simulink model "Shamit_jitesh"  (R2018a)
settings: Solver=VariableStepAuto  StartTime=0.0  StopTime=10.0  RelTol=1e-3
settings Model: Creator=shami  LastModifiedBy=shami

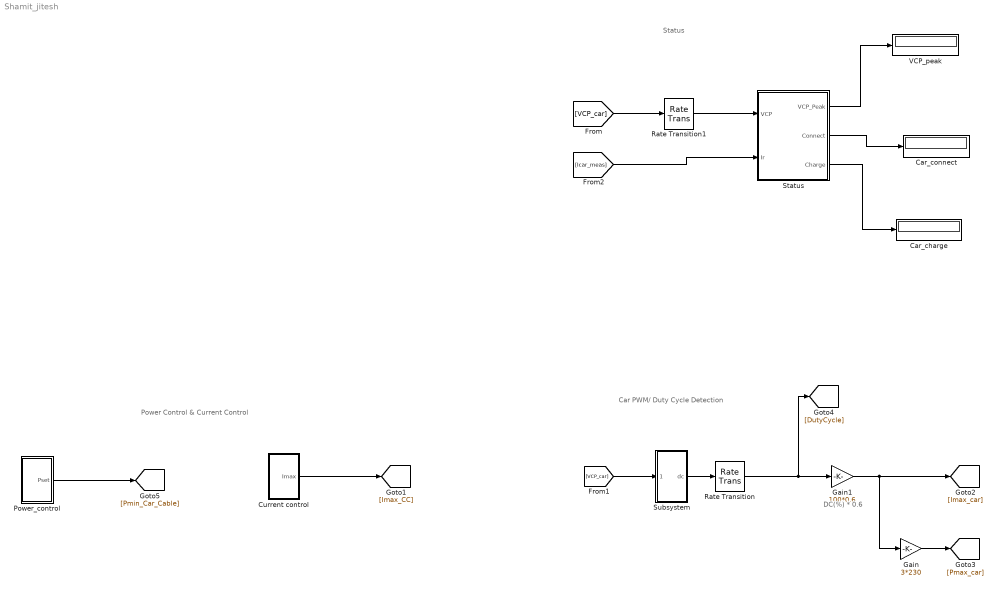
== system Shamit_jitesh ==
  note: Status
  note: Power Control & Current Control
  note: DC(%) * 0.6
  note: Car PWM/ Duty Cycle Detection
  Car_charge : Display
  Car_connect : Display
  Current control : Subsystem
  Gain : Gain  Gain=3*230
  Gain1 : Gain  Gain=100*0.6
  Power_control : Subsystem
  Rate Transition : RateTransition
  Rate Transition1 : RateTransition
  Status : Subsystem
  Subsystem : Subsystem
  VCP_peak : Display
  wires:
  Gain/1 -> [Pmax_car]
  Gain1/1 -> [Imax_car], Gain/1
  [VCP_car] -> Subsystem/1(pwm)
  Subsystem/1(dc) -> Rate Transition/1
  Rate Transition/1 -> [DutyCycle], Gain1/1
  Current control/1(Imax) -> [Imax_CC]
  Power_control/1(Pset) -> [Pmin_Car_Cable]
  [VCP_car] -> Rate Transition1/1
  Status/3("Charge ") -> Car_charge/1
  Status/1(VCP_Peak) -> VCP_peak/1
  [Icar_meas] -> Status/2(Ir)
  Status/2("Connect ") -> Car_connect/1
  Rate Transition1/1 -> Status/1(VCP)

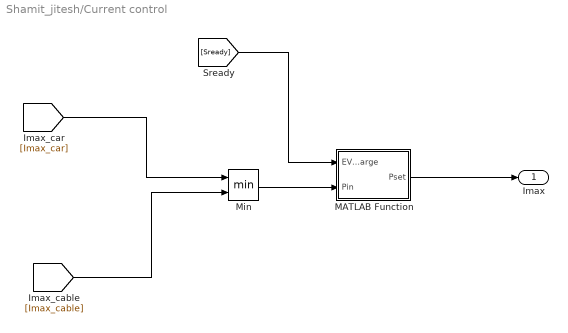
== system Shamit_jitesh/Current control ==
  MATLAB Function : MATLAB Function  TreatAsAtomicUnit=on
  Min : MinMax  Inputs=2
  Imax : Outport
  wires:
  MATLAB Function/1(Pset) -> Imax/1
  Min/1 -> MATLAB Function/2(Pin)
  [Imax_cable] -> Min/2
  [Sready] -> MATLAB Function/1(EV_charge)
  [Imax_car] -> Min/1

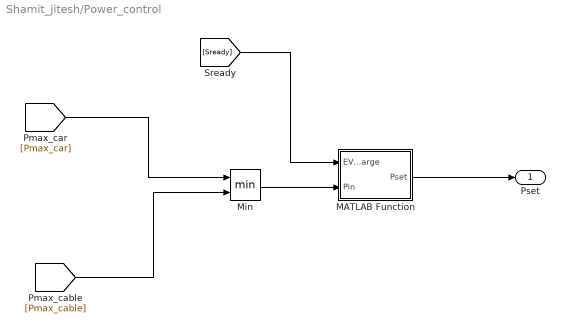
== system Shamit_jitesh/Power_control ==
  MATLAB Function : MATLAB Function  TreatAsAtomicUnit=on
  Min : MinMax  Inputs=2
  Pset : Outport
  wires:
  [Pmax_car] -> Min/1
  Min/1 -> MATLAB Function/2(Pin)
  [Pmax_cable] -> Min/2
  MATLAB Function/1(Pset) -> Pset/1
  [Sready] -> MATLAB Function/1(EV_charge)

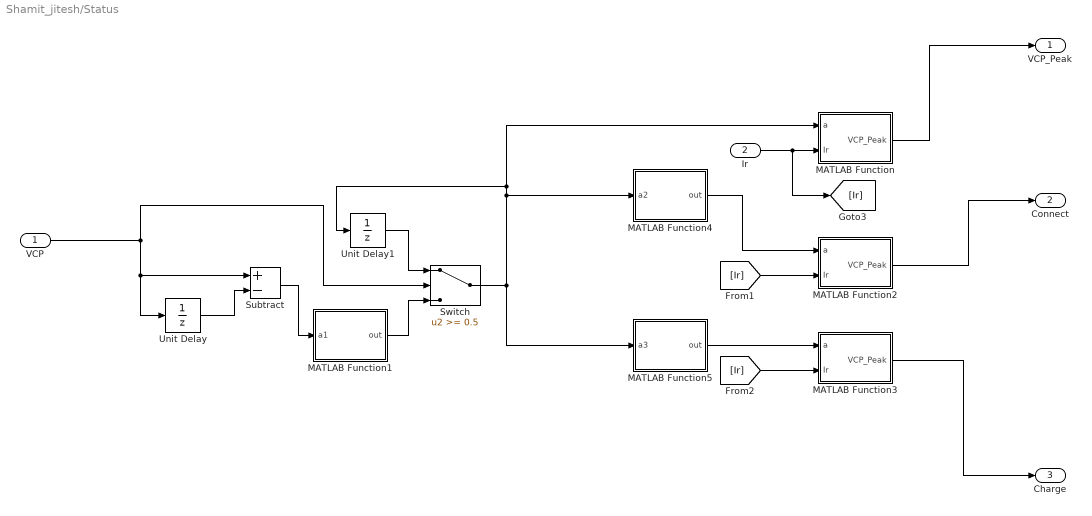
== system Shamit_jitesh/Status ==
  VCP : Inport
  Ir : Inport  Port=2
  MATLAB Function : MATLAB Function  TreatAsAtomicUnit=on
  MATLAB Function1 : MATLAB Function  TreatAsAtomicUnit=on
  MATLAB Function2 : MATLAB Function  TreatAsAtomicUnit=on
  MATLAB Function3 : MATLAB Function  TreatAsAtomicUnit=on
  MATLAB Function4 : MATLAB Function  TreatAsAtomicUnit=on
  MATLAB Function5 : MATLAB Function  TreatAsAtomicUnit=on
  Subtract : Sum  Inputs=+-
  Switch : Switch  Threshold=0.5
  Unit Delay : UnitDelay  SampleTime=-1
  Unit Delay1 : UnitDelay  SampleTime=-1
  VCP_Peak : Outport
  "Connect " : Outport  Port=2
  "Charge " : Outport  Port=3
  wires:
  Switch/1 -> MATLAB Function5/1(a3), MATLAB Function4/1(a2), Unit Delay1/1, MATLAB Function/1(a)
  Unit Delay/1 -> Subtract/2
  Unit Delay1/1 -> Switch/1
  VCP/1 -> Switch/2, Unit Delay/1, Subtract/1
  Subtract/1 -> MATLAB Function1/1(a1)
  MATLAB Function1/1(out) -> Switch/3
  MATLAB Function4/1(out) -> MATLAB Function2/1(a)
  MATLAB Function5/1(out) -> MATLAB Function3/1(a)
  MATLAB Function/1(VCP_Peak) -> VCP_Peak/1
  MATLAB Function2/1(VCP_Peak) -> "Connect "/1
  MATLAB Function3/1(VCP_Peak) -> "Charge "/1
  Ir/1 -> MATLAB Function/2(Ir), [Ir]
  [Ir] -> MATLAB Function2/2(Ir)
  [Ir] -> MATLAB Function3/2(Ir)

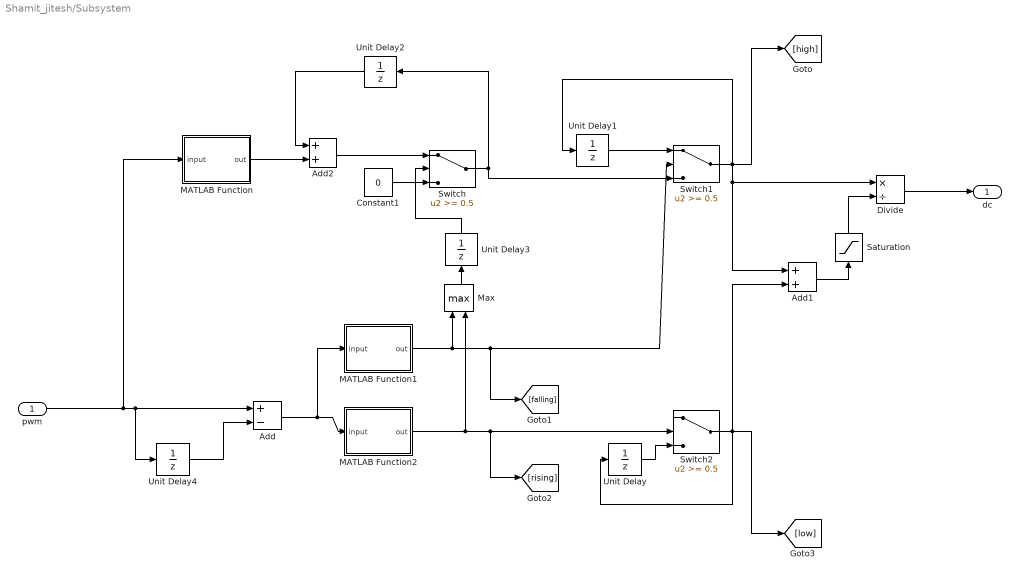
== system Shamit_jitesh/Subsystem ==
  pwm : Inport
  Add : Sum  Inputs=+-
  Add1 : Sum
  Add2 : Sum
  Constant1 : Constant  Value=0
  Divide : Product  Inputs=*/
  MATLAB Function : MATLAB Function  TreatAsAtomicUnit=on
  MATLAB Function1 : MATLAB Function  TreatAsAtomicUnit=on
  MATLAB Function2 : MATLAB Function  TreatAsAtomicUnit=on
  Max : MinMax  Function=max  Inputs=2
  Saturation : Saturate  UpperLimit=inf  LowerLimit=1e-5
  Switch : Switch  Threshold=0.5
  Switch1 : Switch  Threshold=0.5
  Switch2 : Switch  Threshold=0.5
  Unit Delay{,1..4} (5 alike) : UnitDelay  SampleTime=-1
  dc : Outport
  wires:
  Unit Delay4/1 -> Add/2
  pwm/1 -> MATLAB Function/1(input), Unit Delay4/1, Add/1
  Constant1/1 -> Switch/3
  Switch/1 -> Unit Delay2/1, Switch1/3
  Max/1 -> Unit Delay3/1
  Unit Delay1/1 -> Switch1/1
  Switch1/1 -> Unit Delay1/1, [high], Add1/1, Divide/1
  Unit Delay3/1 -> Switch/2
  MATLAB Function1/1(out) -> Switch1/2, [falling], Max/1
  MATLAB Function2/1(out) -> Max/2, [rising], Switch2/2
  Switch2/1 -> Unit Delay/1, [low], Add1/2
  Unit Delay/1 -> Switch2/3
  Add1/1 -> Saturation/1
  Saturation/1 -> Divide/2
  Divide/1 -> dc/1
  Unit Delay2/1 -> Add2/1
  MATLAB Function/1(out) -> Add2/2
  Add2/1 -> Switch/1
  Add/1 -> MATLAB Function1/1(input), MATLAB Function2/1(input)

== matlab function Shamit_jitesh/Subsystem/MATLAB Function1 ==
  data: input input; out output
function out = fcn(input)
int temp = 0;
if(input > -1)
    y = 1;
    int temp = y ; 
    
elseif (input < -1)
    y = 0; 
    int temp = y ; 
    
elseif (input == -1)
    y = temp ;
      
end

out = y;

== matlab function Shamit_jitesh/Subsystem/MATLAB Function ==
  data: input input; out output
function out = fcn(input)
int temp = 0;
if(input > -1000)
    y = 1;
    int temp = y ; 
    
elseif (input < -1000)
    y = 0; 
    int temp = y ; 
    
elseif (input == -1000)
    y = temp ;
      
end

out = y;

== matlab function Shamit_jitesh/Subsystem/MATLAB Function2 ==
  data: input input; out output
function out = fcn(input)
int temp = 0;
if(input > 1)
    y = 1;
    int temp = y ; 
    
elseif (input < 1)
    y = 0; 
    int temp = y ; 
    
elseif (input == 1)
    y = temp ;
      
end

out = y;

== matlab function Shamit_jitesh/Current control/MATLAB Function ==
  data: EV_charge input; Pset output; Pin input
function Pset = fcn(EV_charge, Pin)
if EV_charge == 1
    Pset = Pin;
else
    Pset = 0;
end

== matlab function Shamit_jitesh/Power_control/MATLAB Function ==
  data: EV_charge input; Pset output; Pin input
function Pset = fcn(EV_charge, Pin)
if EV_charge == 1
    Pset = Pin;
else
    Pset = 0;
end

== matlab function Shamit_jitesh/Status/MATLAB Function ==
  data: a input; Ir input; VCP_Peak output
function VCP_Peak = fcn(a, Ir)
int temp = 0;
if(Ir < 1e-6)
    y = 0;
    int temp = y

elseif (Ir > 1e-6)
    y = a;    
    int temp = y;

elseif (Ir == 1e-6)
    y = temp;
end

VCP_Peak = y;

== matlab function Shamit_jitesh/Status/MATLAB Function1 ==
  data: a1 input; out output
function out = fcn(a1)
int temp = 0;
if(a1 > 1)
    y = 1;
    int temp = y;
elseif (a1 < 1)
    y = 0;    
    int temp = y;

elseif (a1 == 1)
    y = temp;
    
end

out = y;

== matlab function Shamit_jitesh/Status/MATLAB Function2 ==
  data: a input; Ir input; VCP_Peak output
function VCP_Peak = fcn(a, Ir)
int temp = 0;
if(Ir < 1e-6)
    y = 0;
    int temp = y

elseif (Ir > 1e-6)
    y = a;    
    int temp = y;

elseif (Ir == 1e-6)
    y = temp;
end

VCP_Peak = y;

== matlab function Shamit_jitesh/Status/MATLAB Function3 ==
  data: a input; Ir input; VCP_Peak output
function VCP_Peak = fcn(a, Ir)
int temp = 0;
if(Ir < 1e-6)
    y = 0;
    int temp = y

elseif (Ir > 1e-6)
    y = a;    
    int temp = y;

elseif (Ir == 1e-6)
    y = temp;
end

VCP_Peak = y;

== matlab function Shamit_jitesh/Status/MATLAB Function4 ==
  data: a2 input; out output
function out = fcn(a2)
int temp = 0;
if(a2 < 9)
    y = 1;  
    int temp = y;
elseif (a2 > 9)
    y = 0;    
    int temp = y;
    
elseif (a2 == 9)
    y = temp;
end

out = y;

== matlab function Shamit_jitesh/Status/MATLAB Function5 ==
  data: a3 input; out output
function out = fcn(a3)
int temp = 0;
if(a3 < 6)
    y = 1;  
    int temp = y;
elseif(a3 > 6)
    y = 0;    
    int temp = y;
    
elseif (a3 == 6)
    y = temp;
          
end

out = y;
